simulink model "LedCount_dir"  (R2014a)
settings: Solver=FixedStepDiscrete  StartTime=0.0  StopTime=400000  FixedStep=1  RelTol=1e-3
libraries: hdlsllib x17, simulink x4
settings Model: Creator=you.r  LastModifiedBy=you.r
settings OptimizationCC: BlockReduction=off  ConditionallyExecuteInputs=off  InlineParams=on
settings DebuggingCC: AlgebraicLoopMsg=error
settings HardwareCC: ProdHWDeviceType=ASIC/FPGA->ASIC/FPGA  ProdEqTarget=off

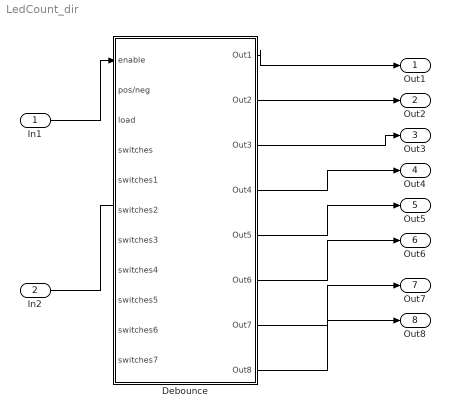
== system LedCount_dir ==
  In1 : Inport  OutDataTypeStr=boolean  SampleTime=1
  In2 : Inport  Port=2  OutDataTypeStr=boolean  SampleTime=1
  Debounce : Subsystem  TreatAsAtomicUnit=on
  Out1 : Outport  SampleTime=1
  Out2 : Outport  Port=2  SampleTime=1
  Out3 : Outport  Port=3  SampleTime=1
  Out4 : Outport  Port=4  SampleTime=1
  Out5 : Outport  Port=5  SampleTime=1
  Out6 : Outport  Port=6  SampleTime=1
  Out7 : Outport  Port=7  SampleTime=1
  Out8 : Outport  Port=8  SampleTime=1
  wires:
  In1/1 -> Debounce/1(enable)
  Debounce/1(Out1) -> Out1/1
  Debounce/2(Out2) -> Out2/1
  Debounce/3(Out3) -> Out3/1
  Debounce/4(Out4) -> Out4/1
  Debounce/5(Out5) -> Out5/1
  Debounce/6(Out6) -> Out6/1
  Debounce/7(Out7) -> Out7/1
  Debounce/8(Out8) -> Out8/1
  In2/1 -> ?

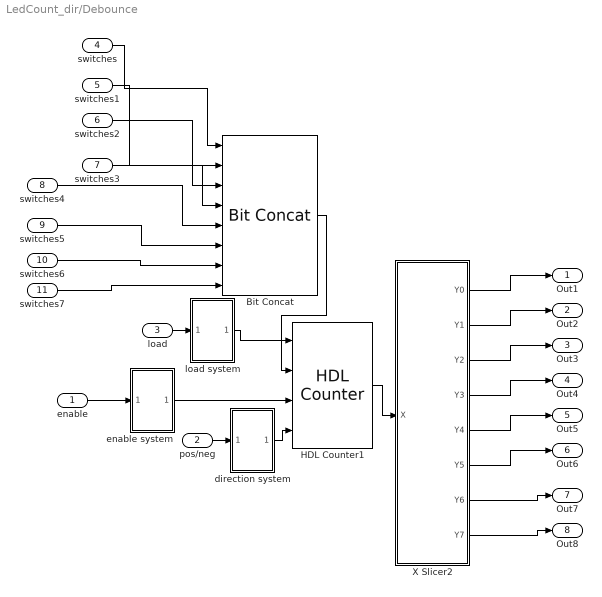
== system LedCount_dir/Debounce ==
  enable : Inport  OutDataTypeStr=boolean  SampleTime=1
  pos/neg : Inport  Port=2  OutDataTypeStr=boolean  SampleTime=1
  load : Inport  Port=3  OutDataTypeStr=boolean  SampleTime=1
  switches : Inport  Port=4  OutDataTypeStr=boolean  SampleTime=1
  switches1 : Inport  Port=5  OutDataTypeStr=boolean  SampleTime=1
  switches2 : Inport  Port=6  OutDataTypeStr=boolean  SampleTime=1
  switches3 : Inport  Port=7  OutDataTypeStr=boolean  SampleTime=1
  switches4 : Inport  Port=8  OutDataTypeStr=boolean  SampleTime=1
  switches5 : Inport  Port=9  OutDataTypeStr=boolean  SampleTime=1
  switches6 : Inport  Port=10  OutDataTypeStr=boolean  SampleTime=1
  switches7 : Inport  Port=11  OutDataTypeStr=boolean  SampleTime=1
  Bit Concat : hdlsllib/HDL Operations/Bit Concat  numInputs=8
  HDL Counter1 : hdlsllib/HDL Operations/HDL Counter  CountType=Count limited  CountInit=0  CountStep=1  CountMax=255  CountFromType=Initial value  CountFrom=0  CountResetPort=off  CountLoadPort=on  CountEnbPort=on  CountDirPort=on  CountDataType=Unsigned  CountWordLen=8  CountFracLen=0  CountSampTime=1
  X Slicer2 : Subsystem
  direction system : Subsystem
  enable system : Subsystem
  load system : Subsystem
  Out1 : Outport  SampleTime=1
  Out2 : Outport  Port=2  SampleTime=1
  Out3 : Outport  Port=3  SampleTime=1
  Out4 : Outport  Port=4  SampleTime=1
  Out5 : Outport  Port=5  SampleTime=1
  Out6 : Outport  Port=6  SampleTime=1
  Out7 : Outport  Port=7  SampleTime=1
  Out8 : Outport  Port=8  SampleTime=1
  wires:
  HDL Counter1/1 -> X Slicer2/1(X)
  X Slicer2/6(Y5) -> Out6/1
  X Slicer2/2(Y1) -> Out2/1
  X Slicer2/7(Y6) -> Out7/1
  X Slicer2/8(Y7) -> Out8/1
  X Slicer2/3(Y2) -> Out3/1
  X Slicer2/4(Y3) -> Out4/1
  X Slicer2/5(Y4) -> Out5/1
  X Slicer2/1(Y0) -> Out1/1
  enable/1 -> enable system/1(In1)
  enable system/1(Out1) -> HDL Counter1/3
  pos/neg/1 -> direction system/1(In1)
  direction system/1(Out1) -> HDL Counter1/4
  switches4/1 -> Bit Concat/5
  switches5/1 -> Bit Concat/6
  switches3/1 -> Bit Concat/4
  switches6/1 -> Bit Concat/7
  switches2/1 -> Bit Concat/3
  switches1/1 -> Bit Concat/2
  switches7/1 -> Bit Concat/8
  switches/1 -> Bit Concat/1
  Bit Concat/1 -> HDL Counter1/2
  load/1 -> load system/1(In1)
  load system/1(Out1) -> HDL Counter1/1

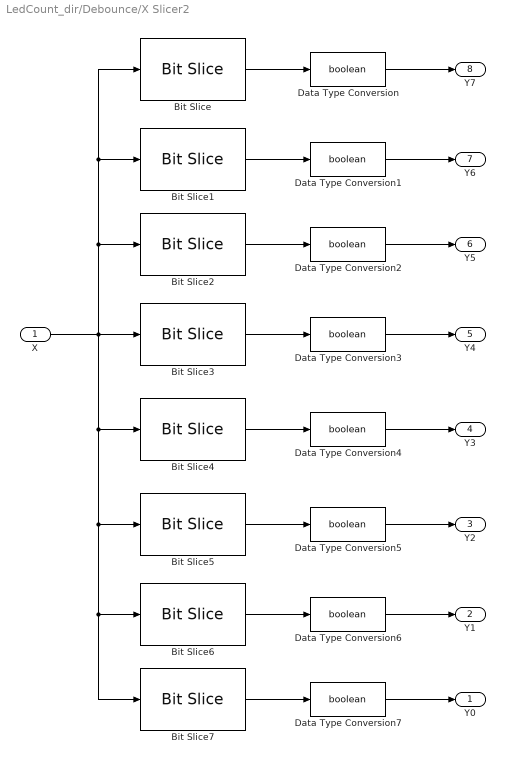
== system LedCount_dir/Debounce/X Slicer2 ==
  X : Inport  OutDataTypeStr=uint8  SampleTime=1
  Bit Slice : hdlsllib/HDL Operations/Bit Slice  lidx=7  ridx=7
  Bit Slice1 : hdlsllib/HDL Operations/Bit Slice  lidx=6  ridx=6
  Bit Slice2 : hdlsllib/HDL Operations/Bit Slice  lidx=5  ridx=5
  Bit Slice3 : hdlsllib/HDL Operations/Bit Slice  lidx=4  ridx=4
  Bit Slice4 : hdlsllib/HDL Operations/Bit Slice  lidx=3  ridx=3
  Bit Slice5 : hdlsllib/HDL Operations/Bit Slice  lidx=2  ridx=2
  Bit Slice6 : hdlsllib/HDL Operations/Bit Slice  lidx=1  ridx=1
  Bit Slice7 : hdlsllib/HDL Operations/Bit Slice  lidx=0  ridx=0
  Data Type Conversion{,1..7} (8 alike) : DataTypeConversion  OutDataTypeStr=boolean
  Y0 : Outport  OutDataTypeStr=boolean  SampleTime=1
  Y1 : Outport  Port=2  OutDataTypeStr=boolean  SampleTime=1
  Y2 : Outport  Port=3  OutDataTypeStr=boolean  SampleTime=1
  Y3 : Outport  Port=4  OutDataTypeStr=boolean  SampleTime=1
  Y4 : Outport  Port=5  OutDataTypeStr=boolean  SampleTime=1
  Y5 : Outport  Port=6  OutDataTypeStr=boolean  SampleTime=1
  Y6 : Outport  Port=7  OutDataTypeStr=boolean  SampleTime=1
  Y7 : Outport  Port=8  OutDataTypeStr=boolean  SampleTime=1
  wires:
  X/1 -> Bit Slice4/1, Bit Slice5/1, Bit Slice6/1, Bit Slice7/1, Bit Slice3/1, Bit Slice2/1, Bit Slice1/1, Bit Slice/1
  Data Type Conversion/1 -> Y7/1
  Data Type Conversion1/1 -> Y6/1
  Bit Slice2/1 -> Data Type Conversion2/1
  Bit Slice3/1 -> Data Type Conversion3/1
  Bit Slice4/1 -> Data Type Conversion4/1
  Data Type Conversion6/1 -> Y1/1
  Bit Slice/1 -> Data Type Conversion/1
  Bit Slice1/1 -> Data Type Conversion1/1
  Bit Slice6/1 -> Data Type Conversion6/1
  Data Type Conversion7/1 -> Y0/1
  Bit Slice7/1 -> Data Type Conversion7/1
  Bit Slice5/1 -> Data Type Conversion5/1
  Data Type Conversion2/1 -> Y5/1
  Data Type Conversion3/1 -> Y4/1
  Data Type Conversion4/1 -> Y3/1
  Data Type Conversion5/1 -> Y2/1

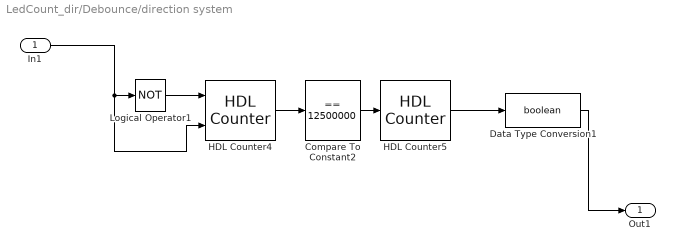
== system LedCount_dir/Debounce/direction system ==
  In1 : Inport
  Compare To Constant2 : simulink/Logic and Bit Operations/Compare To Constant  relop===  const=12500000  OutDataTypeStr=boolean
  Data Type Conversion1 : DataTypeConversion  OutDataTypeStr=boolean
  HDL Counter4 : hdlsllib/HDL Operations/HDL Counter  CountType=Free running  CountInit=0  CountStep=1  CountMax=100  CountFromType=Initial value  CountFrom=0  CountResetPort=on  CountLoadPort=off  CountEnbPort=on  CountDirPort=off  CountDataType=Unsigned  CountWordLen=32  CountFracLen=0  CountSampTime=1
  HDL Counter5 : hdlsllib/HDL Operations/HDL Counter  CountType=Count limited  CountInit=0  CountStep=1  CountMax=1  CountFromType=Initial value  CountFrom=0  CountResetPort=off  CountLoadPort=off  CountEnbPort=on  CountDirPort=off  CountDataType=Unsigned  CountWordLen=1  CountFracLen=0  CountSampTime=1
  Logical Operator1 : Logic  Operator=NOT  IconShape=distinctive  AllPortsSameDT=off  OutDataTypeStr=boolean  SampleTime=1
  Out1 : Outport
  wires:
  Data Type Conversion1/1 -> Out1/1
  In1/1 -> HDL Counter4/2, Logical Operator1/1
  Logical Operator1/1 -> HDL Counter4/1
  HDL Counter4/1 -> Compare To Constant2/1
  HDL Counter5/1 -> Data Type Conversion1/1
  Compare To Constant2/1 -> HDL Counter5/1

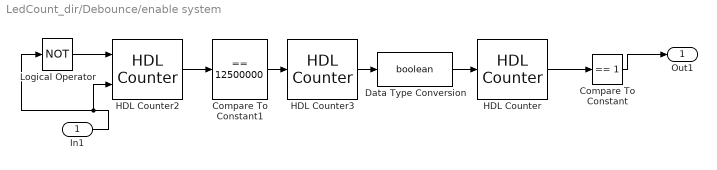
== system LedCount_dir/Debounce/enable system ==
  In1 : Inport
  Compare To Constant : simulink/Logic and Bit Operations/Compare To Constant  relop===  const=1  OutDataTypeStr=boolean
  Compare To Constant1 : simulink/Logic and Bit Operations/Compare To Constant  relop===  const=12500000  OutDataTypeStr=boolean
  Data Type Conversion : DataTypeConversion  OutDataTypeStr=boolean
  HDL Counter : hdlsllib/HDL Operations/HDL Counter  CountType=Count limited  CountInit=0  CountStep=1  CountMax=25000000  CountFromType=Initial value  CountFrom=0  CountResetPort=off  CountLoadPort=off  CountEnbPort=on  CountDirPort=off  CountDataType=Unsigned  CountWordLen=32  CountFracLen=0  CountSampTime=1
  HDL Counter2 : hdlsllib/HDL Operations/HDL Counter  CountType=Free running  CountInit=0  CountStep=1  CountMax=100  CountFromType=Initial value  CountFrom=0  CountResetPort=on  CountLoadPort=off  CountEnbPort=on  CountDirPort=off  CountDataType=Unsigned  CountWordLen=32  CountFracLen=0  CountSampTime=1
  HDL Counter3 : hdlsllib/HDL Operations/HDL Counter  CountType=Count limited  CountInit=0  CountStep=1  CountMax=1  CountFromType=Initial value  CountFrom=0  CountResetPort=off  CountLoadPort=off  CountEnbPort=on  CountDirPort=off  CountDataType=Unsigned  CountWordLen=1  CountFracLen=0  CountSampTime=1
  Logical Operator : Logic  Operator=NOT  IconShape=distinctive  AllPortsSameDT=off  OutDataTypeStr=boolean  SampleTime=1
  Out1 : Outport
  wires:
  Compare To Constant/1 -> Out1/1
  HDL Counter/1 -> Compare To Constant/1
  In1/1 -> Logical Operator/1, HDL Counter2/2
  Logical Operator/1 -> HDL Counter2/1
  HDL Counter2/1 -> Compare To Constant1/1
  HDL Counter3/1 -> Data Type Conversion/1
  Compare To Constant1/1 -> HDL Counter3/1
  Data Type Conversion/1 -> HDL Counter/1

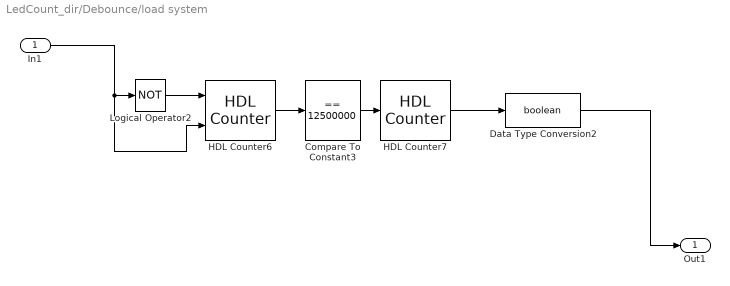
== system LedCount_dir/Debounce/load system ==
  In1 : Inport
  Compare To Constant3 : simulink/Logic and Bit Operations/Compare To Constant  relop===  const=12500000  OutDataTypeStr=boolean
  Data Type Conversion2 : DataTypeConversion  OutDataTypeStr=boolean
  HDL Counter6 : hdlsllib/HDL Operations/HDL Counter  CountType=Free running  CountInit=0  CountStep=1  CountMax=100  CountFromType=Initial value  CountFrom=0  CountResetPort=on  CountLoadPort=off  CountEnbPort=on  CountDirPort=off  CountDataType=Unsigned  CountWordLen=32  CountFracLen=0  CountSampTime=1
  HDL Counter7 : hdlsllib/HDL Operations/HDL Counter  CountType=Count limited  CountInit=0  CountStep=1  CountMax=1  CountFromType=Initial value  CountFrom=0  CountResetPort=off  CountLoadPort=off  CountEnbPort=on  CountDirPort=off  CountDataType=Unsigned  CountWordLen=1  CountFracLen=0  CountSampTime=1
  Logical Operator2 : Logic  Operator=NOT  IconShape=distinctive  AllPortsSameDT=off  OutDataTypeStr=boolean  SampleTime=1
  Out1 : Outport
  wires:
  HDL Counter6/1 -> Compare To Constant3/1
  Data Type Conversion2/1 -> Out1/1
  In1/1 -> HDL Counter6/2, Logical Operator2/1
  Logical Operator2/1 -> HDL Counter6/1
  HDL Counter7/1 -> Data Type Conversion2/1
  Compare To Constant3/1 -> HDL Counter7/1
